simulink model "formationSim"  (R2021a)
settings: Solver=VariableStepAuto  StartTime=0.0  StopTime=10.0  RelTol=1e-3
undefined symbols (not defined in the file): B, barrier, d, epsilon, gamma, O, params, R, u0, x0
libraries: simulink x2
settings Model: Creator=sylva  LastModifiedBy=antonioterpin
settings SolverCC: AlgebraicLoopSolver=TrustRegion
settings DebuggingCC: SFMachineParentedDataDiag=warning

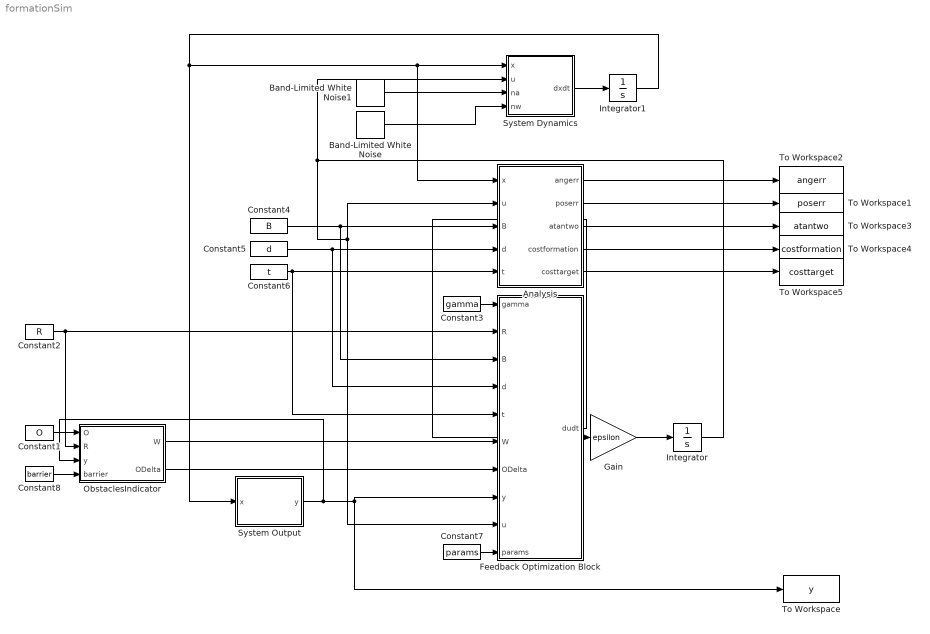
== system formationSim ==
  Analysis : MATLAB Function  TreatAsAtomicUnit=on
  Band-Limited White Noise : simulink/Sources/Band-Limited White Noise  Cov=0  Ts=0.1  seed=[23341]
  Band-Limited White Noise1 : simulink/Sources/Band-Limited White Noise  Cov=0  Ts=0.1  seed=[23341]
  Constant1 : Constant  Value=O  VectorParams1D=off
  Constant2 : Constant  Value=R  VectorParams1D=off
  Constant3 : Constant  Value=gamma  VectorParams1D=off
  Constant4 : Constant  Value=B  VectorParams1D=off
  Constant5 : Constant  Value=d  VectorParams1D=off
  Constant6 : Constant  Value=t  VectorParams1D=off
  Constant7 : Constant  Value=params  VectorParams1D=off
  Constant8 : Constant  Value=barrier  VectorParams1D=off
  Feedback Optimization Block : MATLAB Function  TreatAsAtomicUnit=on
  Gain : Gain  Gain=epsilon
  Integrator : Integrator  InitialCondition=u0
  Integrator1 : Integrator  InitialCondition=x0
  ObstaclesIndicator : MATLAB Function  TreatAsAtomicUnit=on
  System Dynamics : MATLAB Function  TreatAsAtomicUnit=on
  System Output : MATLAB Function  TreatAsAtomicUnit=on
  To Workspace : ToWorkspace  VariableName=y  SaveFormat=Timeseries  SampleTime=-1
  To Workspace1 : ToWorkspace  VariableName=poserr  SaveFormat=Timeseries  SampleTime=-1
  To Workspace2 : ToWorkspace  VariableName=angerr  SaveFormat=Timeseries  SampleTime=-1
  To Workspace3 : ToWorkspace  VariableName=atantwo  SaveFormat=Timeseries  SampleTime=-1
  To Workspace4 : ToWorkspace  VariableName=costformation  SaveFormat=Timeseries  SampleTime=-1
  To Workspace5 : ToWorkspace  VariableName=costtarget  SaveFormat=Timeseries  SampleTime=-1
  wires:
  Constant2/1 -> ObstaclesIndicator/2(R), Feedback Optimization Block/2(R)
  Constant5/1 -> Feedback Optimization Block/4(d), Analysis/4(d)
  Constant6/1 -> Feedback Optimization Block/5(t), Analysis/5(t)
  Integrator/1 -> Feedback Optimization Block/9(u), Analysis/2(u), System Dynamics/2(u)
  Feedback Optimization Block/1(dudt) -> Gain/1
  Integrator1/1 -> Analysis/1(x), System Dynamics/1(x), System Output/1(x)
  System Dynamics/1(dxdt) -> Integrator1/1
  Constant1/1 -> ObstaclesIndicator/1(O)
  ObstaclesIndicator/2(ODelta) -> Feedback Optimization Block/7(ODelta)
  System Output/1(y) -> Feedback Optimization Block/8(y), To Workspace/1, ObstaclesIndicator/3(y)
  Constant8/1 -> ObstaclesIndicator/4(barrier)
  Analysis/2(poserr) -> To Workspace1/1
  Band-Limited White Noise1/1 -> System Dynamics/3(na)
  Analysis/1(angerr) -> To Workspace2/1
  ObstaclesIndicator/1(W) -> Feedback Optimization Block/6(W)
  Analysis/5(costtarget) -> To Workspace5/1
  Gain/1 -> Integrator/1
  Band-Limited White Noise/1 -> System Dynamics/4(nw)
  Analysis/4(costformation) -> To Workspace4/1
  Constant7/1 -> Feedback Optimization Block/10(params)
  Constant4/1 -> Feedback Optimization Block/3(B), Analysis/3(B)
  Constant3/1 -> Feedback Optimization Block/1(gamma)
  Analysis/3(atantwo) -> To Workspace3/1

== matlab function formationSim/Feedback Optimization Block ==
  data: gamma input; R input; B input; d input; t input; W input; ODelta input; y input; u input; dudt output; params input
function dudt = ctrl(gamma, R, B, d, t, W, ODelta, y, u, params)
dudt = ctrl_implemented(gamma, R, B, d, t, W, ODelta, y, u, params);
end

== matlab function formationSim/System Dynamics ==
  data: x input; u input; dxdt output; na input; nw input
function dxdt = dyn(x, u, na, nw)
dxdt = dyn_implemented_velocity(x, u, na, nw);
end

== matlab function formationSim/System Output ==
  data: x input; y output
function y = out(x)
y = out_implemented(x);
end

== matlab function formationSim/ObstaclesIndicator ==
  data: W output; O input; R input; y input; ODelta output; barrier input
function [W,ODelta] = obst(O,R,y,barrier)
[W,ODelta] = obst_implemented(O,R,y,barrier);
end

== matlab function formationSim/Analysis ==
  data: x input; angerr output; u input; poserr output; atantwo output; B input; d input; t input; costformation output; costtarget output
function [angerr,poserr,atantwo,costformation,costtarget] = analysis(x,u,B,d,t)
x = reshape(x,3,[]);
u = reshape(u,2,[]);
y = reshape(x(1:2,:),[],1);
delta = u - x(1:2,:);
poserr = vecnorm(delta);
atantwo = atan2(delta(2,:),delta(1,:));
angerr = atantwo - x(3,:);
costformation = .5 * sum((kron(B, eye(2)).' * y - d(:)).^2);
costtarget = .5 * sum((y - repmat(t, size(x,2), 1)).^2);
end
